simulink model "m0807163636"  (R2023b)
settings: Solver=FixedStepDiscrete  StartTime=0.0  StopTime=inf  FixedStep=0.01  RelTol=1e-3
settings Model: Creator=developer  LastModifiedBy=developer
settings DataIOCC: SaveFormat=StructureWithTime  ReturnWorkspaceOutputs=off
settings OptimizationCC: EnhancedBackFolding=on  OptimizeBlockOrder=speed  DifferentSizesBufferReuse=on  OptimizationCustomize=off
settings DebuggingCC: ParameterTunabilityLossMsg=error  UnconnectedInputMsg=warning  UnconnectedOutputMsg=warning  UnconnectedLineMsg=warning  ArithmeticOperatorsInVariantConditions=warning
settings ModelReferenceCC: ModelReferenceNumInstancesAllowed=Single
settings SFSimCC: MATLABDynamicMemAlloc=off  CustomCodeUndefinedFunction=UseInterfaceOnly

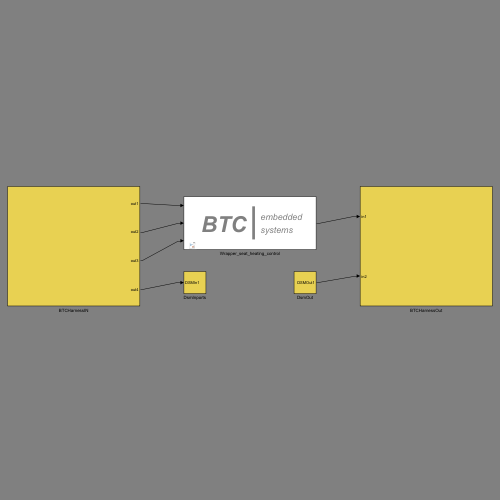
[thumbnail: Simulink's stored preview of the top-level diagram]
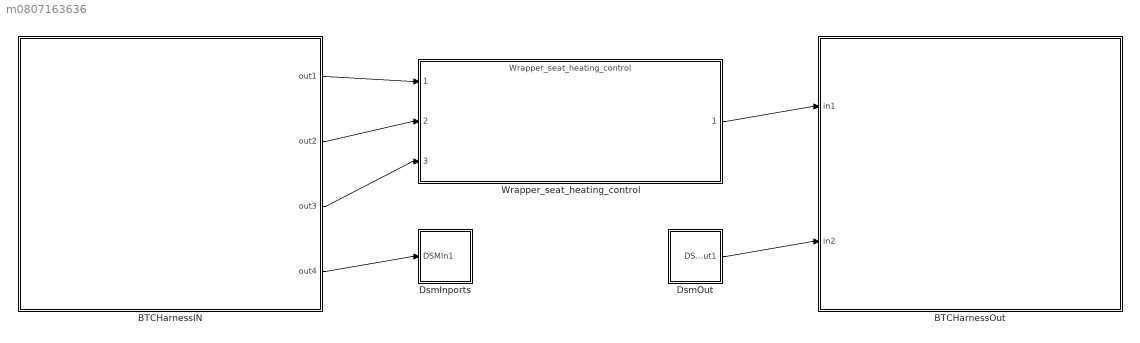
== system m0807163636 ==
  BTCHarnessIN : Subsystem  Priority=100
  BTCHarnessOut : Subsystem  Priority=500
  DsmInports : Subsystem  Priority=200
  DsmOut : Subsystem  Priority=400
  Wrapper_seat_heating_control : ModelReference  Priority=300  ModelNameDialog=Wrapper_seat_heating_control.slx  SimulationMode=Normal  ModelReferenceVersion=1.1
      mask Display: disp('\color{gray}\it\fontsize{20}                          embedded\newline                          systems', 'texmode', 'on');disp('{{\color{gray}\bf\fontsize{50}\it   BTC}  \fontsize{80}|      \color{black}\fontsize{20}\newline }', 'texmode', 'on');
  wires:
  BTCHarnessIN/1(out1) -> Wrapper_seat_heating_control/1
  BTCHarnessIN/2(out2) -> Wrapper_seat_heating_control/2
  BTCHarnessIN/3(out3) -> Wrapper_seat_heating_control/3
  BTCHarnessIN/4(out4) -> DsmInports/1(DSMIn1)
  Wrapper_seat_heating_control/1 -> BTCHarnessOut/1(in1)
  DsmOut/1(DSMOut1) -> BTCHarnessOut/2(in2)

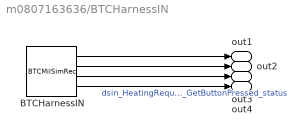
== system m0807163636/BTCHarnessIN ==
  BTCHarnessIN : S-Function  Tag=BTC_SIM_MODEL_INPUTS  FunctionName=BTCMilSimRec  Parameters='HarnessModelIn_1723041396532.xml','',''  SFunctionDeploymentMode=off  EnableBusSupport=off
  out1 : Outport
  out2 : Outport  Port=2
  out3 : Outport  Port=3
  out4 : Outport  Port=4
  wires:
  BTCHarnessIN/1 -> out1/1
  BTCHarnessIN/2 -> out2/1
  BTCHarnessIN/3 -> out3/1
  BTCHarnessIN/4 -> out4/1  "dsin_HeatingRequest_GetButtonPressed_status"

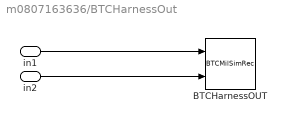
== system m0807163636/BTCHarnessOut ==
  in1 : Inport
  in2 : Inport  Port=2
  BTCHarnessOUT : S-Function  Tag=BTC_SIM_MODEL_OUTPUTS  FunctionName=BTCMilSimRec  Parameters='HarnessModelOut_1723041396532.xml','',''  SFunctionDeploymentMode=off  EnableBusSupport=off
  wires:
  in1/1 -> BTCHarnessOUT/1
  in2/1 -> BTCHarnessOUT/2

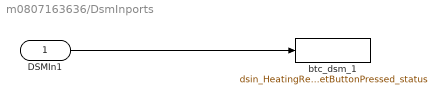
== system m0807163636/DsmInports ==
  DSMIn1 : Inport
  btc_dsm_1 : DataStoreWrite  DataStoreName=dsin_HeatingRequest_GetButtonPressed_status  IndexOptions=Index vector (dialog)  Indices=1  OutputSizes=1
  wires:
  DSMIn1/1 -> btc_dsm_1/1

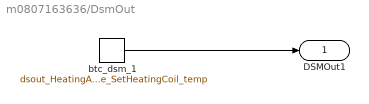
== system m0807163636/DsmOut ==
  btc_dsm_1 : DataStoreRead  DataStoreName=dsout_HeatingActivate_SetHeatingCoil_temp  IndexOptions=Index vector (dialog)  Indices=1  OutputSizes=1
  DSMOut1 : Outport
  wires:
  btc_dsm_1/1 -> DSMOut1/1
